simulink model "c28069_externalSin_T"  (R2018b)
settings: Solver=ode4  StartTime=0.0  StopTime=inf  FixedStep=Ts  RelTol=1e-3
InitFcn:
  | Ts=1e-4
undefined symbols (not defined in the file): serial
libraries: instrumentlib x3
settings Model: Creator=matti  LastModifiedBy=matti
settings HardwareCC: ProdBitPerPointer=32  ProdBitPerSizeT=32  ProdBitPerPtrDiffT=32  ProdWordSize=32  ProdHWDeviceType=Intel->x86-32 (Windows32)
settings SFSimCC: SimUseLocalCustomCode=off
settings RTWCC: RTWUseLocalCustomCode=off
settings CodeAppCC: StateflowObjectComments=on
settings SimscapeCC: SimscapeNormalizeSystem=off

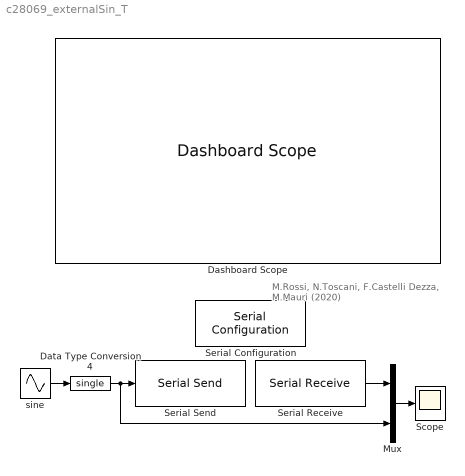
== system c28069_externalSin_T ==
  note: M.Rossi, N.Toscani, F.Castelli Dezza, M.Mauri (2020)
  Dashboard Scope : DashboardScope  WebBlockId=52  TimeSpan=30  Ymin=0  Ymax=2
  Data Type Conversion4 : DataTypeConversion  OutDataTypeStr=single
  Mux : Mux  Inputs=2
  Scope : Scope
  Serial Configuration : instrumentlib/Serial Configuration  Priority=-200000  ComPortMenu=<Please select a port...>  ComPort=COM14  ObjConstructor=serial('COM14');  BaudRate=115200  DataBits=8  Parity=none  StopBits=1  FlowControl=none  Timeout=10  ByteOrder=LittleEndian
  Serial Receive : instrumentlib/Serial Receive  ComPortMenu=<Please select a port...>  ComPort=COM14  ObjConstructor=serial('COM14');  Terminator=<none>  DataSize="[1  1]"  DataType=single  EnableBlockingMode=on  ActionDataUnavailable=Output last received value  CustomValue=0  SampleTime=0.01
  Serial Send : instrumentlib/Serial Send  ComPortMenu=<Please select a port...>  ComPort=COM14  ObjConstructor=serial('COM14');  Terminator=<none>  EnableBlockingMode=on
  sine : Sin  SineType=Sample based  Amplitude=0.5  Bias=0.5  Samples=100  SampleTime=0.1
  wires:
  Mux/1 -> Scope/1
  sine/1 -> Data Type Conversion4/1
  Data Type Conversion4/1 -> Mux/2, Serial Send/1
  Serial Receive/1 -> Mux/1
